simulink model "Ford_T3T6_ArchCnctnDigrm"  (R2016b)
settings: Solver=FixedStepDiscrete  StartTime=0.0  StopTime=10.0  RelTol=1e-3  EnableMultiTasking=on
libraries: canmsglib x15
(part 8 of 15)

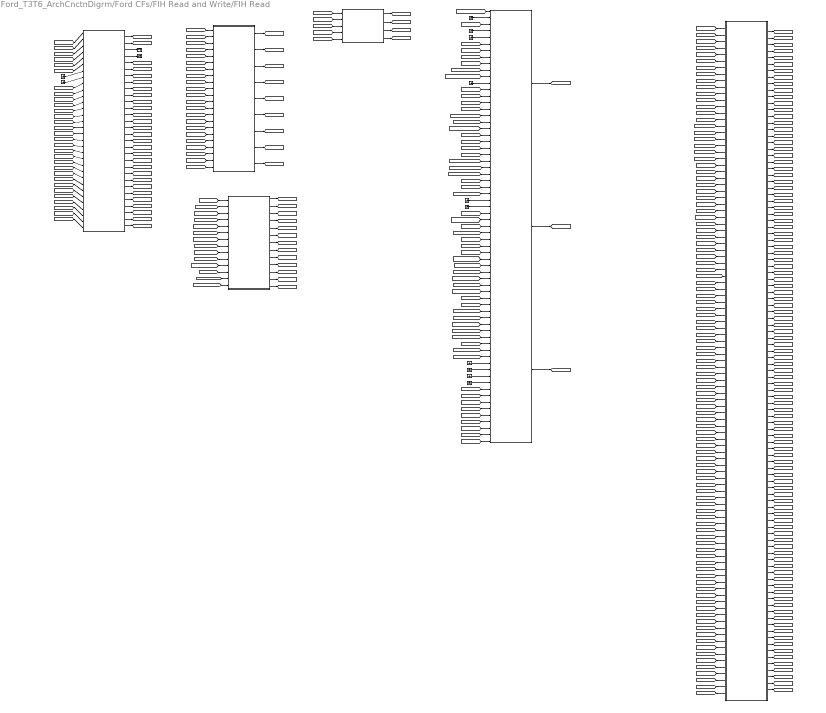
== system Ford_T3T6_ArchCnctnDigrm/Ford CFs/FIH Read and Write/FIH Read ==
  note: ASIL B FIH
  note: ASIL B FIH
  note: ASIL B FIH
  note: ASIL B FIH
  note: ASIL B FIH
  note: ASIL B FIH
  note: FIH_Read_Signal_Status
  note: Enable Disable Feature via DID
  note: Missing in component Req
  note: Bit 2
  note: Status 2 Bit 0
  note: Bit 3
  note: Bit 1
  note: Bit 0
  note: Bit31
  note: Bit24
  note: MM092
  note: Status 2
      | Bit 0 AccelPedalPosValid
      | Bit 1 EngineRPMValid
      | Bit 2 GearLeverPosValid
      | Bit 3 IgnitionStatusValid
      | Bit 4 LSMCBrakeSupportValid
      | Bit 5 PAMStatusValid
      | Bit 6 TBAAvailableValid
      | Bit 7 TBACancelRequestValid
      | Bit 8 TBAEnableValid
      | Bit 9 TBAHitchAngleValid
      | Bit 10 TBAHitchRateValid
      | Bit 11 TBAKnobPositionValid
      | Bit 12 TBAKnobValid
      | Bit 13 TBAMeasurementValid
      | Bit 14 TBATargetValid
      | Bit 15 TBATrackStateValid
      | Bit 16 TBAYawRateValid
      | Bit 17 TBAReverseValid
      | Bit 18 TBAModeRequestValid
      | Bit 19 BrakePedalValid
      | Bit 20-31 NOT USED
  note: Status 1
      | Bit 0 VehicleSpeedValid
      | Bit 1 BrakeTorqueValid
      | Bit 2 VertAccelValid
      | Bit 3 FLWheelCountDirValid
      | Bit 4 FLWheelSpeedValid
      | Bit 5 FRWheelCountDirValid
      | Bit 6 FRWheelSpeedValid
      | Bit 7 LA_IPMAValid
      | Bit 8 LatAccelValid
      | Bit 9 LATCTL_IPMAValid
      | Bit 10 SDMChassisValid
      | Bit 11 PropTorqueValid
      | Bit 12 ReverseGearValid
      | Bit 13 RLWheelCountDirValid
      | Bit 14 RLWheelSpeedValid
      | Bit 15 RRWheelCountDirValid
      | Bit 16 RRWheelSpeedValid
      | Bit 17 SPAOffsetValid
      | Bit 18 TurnSignalValid
      | Bit 19 FilteredVehicleSpeedValid
      | Bit 20 YawRateValid
      | Bit 21 YawRateRawValid
      | Bit 22 YawStabilityValid
      | Bit 23 LongAccelValid
      | Bit 24 ABS_ESC_StatusValid
      | Bit 25 ESA_IPCValid
      | Bit 26 ESA_IPMAValid
      | Bit 27 VehicleSpeedOverGroundValid
      | Bit 28 SPAVelocityValid
      | Bit 29 RelativeSPAValid
      | Bit 30 InputTorqueRawValid
      | Bit 31 AppliedFinalMotorTorqueValid
  note: Add FIH_Read_TBA_EAC_Status()
  note: Add FIH_Read_TBA_EAC_Status() EAC_Status
      | (ExtAgCtrlStsInt)
  note: FIH_Read_APA_Torque_Filtered() APA_Torque_Filtered
      | FIH_Read_EngineSize() EngineTorqueClass
      | FIH_Read_SAPPAngleControlStat1() SAPPAngleControlStat1
      | FIH_Read_SAPPAngleControlStat2() SAPPAngleControlStat2
      | FIH_Read_SAPPAngleControlStat3() SAPPAngleControlStat3
      | FIH_Read_SAPPAngleControlStat4() SAPPAngleControlStat4
      | FIH_Read_SAPPAngleControlStat5() SAPPAngleControlStat5
      | FIH_Read_TBA_EAC_Status() EAC_Status
  note: FIH_Read_EPS_System_Time() SystemTime
      | FIH_Read_WheelBase() VehicleWheelBase
      | FIH_Read_RackPinionRatio() RacktoPinionRatio
      | FIH_Read_VehicleSteeringRatio() VehicleSteeringRatio
      | FIH_Read_EPS_InputTorqueRaw() InputTorqueRaw
      | FIH_Read_EPS_InputTorqueFilt() BCInputTorque
      | FIH_Read_EPS_Assist_Torque() BCAssistTorque
      | FIH_Read_EPS_SteeringAngle() CompensatedSPA
      | FIH_Read_EPS_CompSPA_QF() CompensatedSPAQualityFactor
      | FIH_Read_EPS_ColumnVelocity() SPAVelocity
      | FIH_Read_EPS_VehicleSpeed() FilteredVehicleSpeed
      | FIH_Read_EPS_VehicleSpeed_Raw() VehicleSpeed
      | FIH_Read_TireCircumference() TireCircumference
      | FIH_Read_EPS_Final_Motor_Tq_Rq() RequestedFinalMotorTorque
      | FIH_Read_EPS_Final_Motor_Tq_App() AppliedFinalMotorTorque
      | FIH_Read_EPS_Rel_SteeringAngle() RelativeSPA
      | FIH_Read_EPS_Personalization() SDM_SteeringMode
      | FIH_Read_AngleControlState() INTAngleControlStat1
      | FIH_Read_EPSSystemState() EPSSystemState
      | FIH_Read_MaxAssistanceTorque() MaxAssistanceTorque
  note: To be deleted
  note: To be deleted
  note: CF100
  note: CF100
  note: MMs Does not exist yet
  note: Use FordVehYawRateSnsrIdyHi and FordVehYawRateSnsrIdyLo from MM082
      | and combine them
  note: Should it be FordVehSpdBrkModlVld ??
  note: SDM_SteeringMode
  note: s8p7
  note: U-8
  note: U-32
  note: U-32
  note: U-32
  note: U-32
  note: U-32
  note: U-32
  note: U-32
  note: U-32
  note: U-32
  note: U-16
  note: VehVertComp_A_Actl
  note: GearRvrse_D_Actl
  note: Msg 60A,B,C,D
      | Not available
  note: HSCAN_In4_High
  note: HSCAN_In4_Low
  note: HSCAN_In3_High
  note: HSCAN_In3_Low
  note: HSCAN_In2_High
  note: HSCAN_In2_Low
  note: HSCAN_In1_High
  note: HSCAN_In1_Low
  note: TrlrYaw_W_Actl_D_Qf
  note: TrlrYaw_W_Actl
  note: TrlrIdType_D_Stat
  note: TrlrRvrse_D_Stat
  note: TrlrRvrseMsgTxt_D2_Rq
  note: TrlrHitchYaw_D_Stat
  note: TrlrRvrseEnbl_D2_Stat
  note: TrlrRvrseCancl_B_Rq
  note: TrlrLampCnnct_B_Actl
  note: TrlrAidTrgtId_No_Actl
  note: TrlrHitYaw_AnRate_Actl
  note: TrlrHitchYaw_An_Actl
  note: TrlrBrkActCnnct_B_Actl
  note: HitchToVehAxle_L_Calc
  note: TrlrAxleToBmpr_L_Actl
  note: TrlrAid_D2_Stat
  note: TrlrAidSetup_D2_Rq
  note: TrlrAidEnbl_D2_Rq
  note: TrlrAidMde_D_Rq
  note: TrlrAidCtl_U_RqDrv
  note: TrlrAidSwtch_D_RqDrv
  note: TrlrId_No_Actl
  note: TrlrHitYaw_AnRate_Actl
  note: msg45A
  note: TrlrAnOffstDir_D_Mem
  note: TrlrAid_An3_Actl
  note: TrlrAidCancl_B_Rq
  note: VehVTrlrAid_B_Avail
  note: Msg 459
  note: TrlrTrgtAcquire_D_Stat
  note: Veh_V_ActlBrk
  note: YawStabilityIndex
  note: u-48
  note: Ford_TrlrSnsId_No_Act
  note: VehYaw_W_Actl
  note: VehYawComp_W_Actl
  note: Ford_VehOverGnd_V_Est
  note: Ford_VehLongComp_A_Actl
  note: Ford_VehLatComp_A_Actl
  note: TurnLghtSwtch_D_Stat
  note: Ford_GearPos_D_Actl
  note: TrnRng_D_Rq
  note: CmbbObjColl_T_Actl
  note: EsaOn_B_Rq
  note: CmbbObjRelLong_V_Actl
  note: CmbbObjRelLat_V_Actl
  note: WhlRl_W_Meas
  note: WhlRotatRl_No_Cnt
  note: WhlDirRl_D_Actl
  note: PrplWhlTot2_Tq_Actl
  note: ApaSys_D_Stat
  note: CmbbObjClass_D_Stat
  note: CmbbObjConfdnc_D_Stat
  note: Ford_LsmcBrkDecel_D_Stat1
  note: LaRefAng_No_Req
  note: LaCurvature_No_Calc
  note: CmbbObjDistLong_L_Actl
  note: CmbbObjDistLat_L_Actl
  note: Change source name
  note: LatCtl_D_Rq
  note: LatCtlPrecision_D_Rq
  note: LatCtlPathOffst_L_Actl
  note: LatCtlPath_An_Actl
  note: LatCtlCurv_NoRate_Actl
  note: LatCtlCurv_No_Actl
  note: GearLvrPos_D_Actl
  note: WhlFr_W_Meas
  note: WhlRotatFr_No_Cnt
  note: WhlDirFr_D_Actl
  note: WhlFl_W_Meas
  note: WhlDirFl_D_Actl
  note: EngAout_N_Actl
  note: StabCtlBrkActv_B_Actl
  note: CmbbBrkDis_B_Actl
  note: CmbbDeny_B_ActlBrk
  note: Ignition_Status1
  note: BpedDrvAppl_D_Qf
  note: BpedDrvAppl_D_Actl
  note: StePinOffst_D_Stat1
  note: StePinOffst_An_Est
  note: AbsActv_B_Actl
  note: BrkTot_Tq_Actl
  note: ApedPosPcActl_D_Qf
  note: ApedPos_Pc_ActlArb
  note: LaRampType_B_Req
  note: LatCtlRng_L_Max
  note: LatCtlRampType_D_Rq
  note: HandsOffCnfm_B_Rq
  note: Called by FIH
  note: Called by FIH
  note: Called by FIH
  note: Called by FIH
  note: LkaActvStats_D2_Req
  note: LdwActvStats_D_Req
  note: LdwActvIntns_D_Req
  note: WhlRotatFl_No_Cnt
  note: EsaEnbl_D2_Rq
  note: TireCircumference
      | mm
      | U-16
      | 1
  note: PDC_InternalStatus
      | Table
      | U-32
      |
      | LDW_InternalStatus
      | Table
      | U-32
      |
      | LKA_InternalStatus
      | Table
      | U-32
      |
      | ANC_InternalStatus
      | Table
      | U-32
      |
      | STDR_InternalStatus
      | Table
      | U-32
      |
      | ESA_InternalStatus
      | Table
      | U-32
      |
      | LATCTL_InternalStatus
      | Table
      | U-32
      |
      | TBA_InternalStatus
      | Table
      | U-32
  note: INTAngleControlStat1
      | Table
      | U-8
      |
      | SAPPAngleControlStat1
      | Table
      | U-8
      |
      | SAPPAngleControlStat2
      | No Units
      | Bool
      |
      | SAPPAngleControlStat3
      | No Units
      | Bool
      |
      | SAPPAngleControlStat4
      | No Units
      | Bool
      |
      | SAPPAngleControlStat5
      | No Units
      | Bool
      |
      | SAPPAngleControlStat6
      | No Units
      | Bool
  note: ANC_Diagnostic_Status
      | Table
      | U-8
      |
      | LDW_Diagnostic_Status
      | Table
      | U-8
  note: From DID
  note: // Read --> The Vehicle Physical Parameters (e.g. Wheelbase, Rack-to-Pinion Ratio, etc.) must be provided by Base EPS to In-House Features via Software
      | Read Functions. In-House Features that require these parameters will request it once during Initialization.
  note: WhlRr_W_Meas
  note: WhlRotatRr_No_Cnt
  note: WhlDirRr_D_Actl
  note: To be deleted
  note: To be deleted
  note: To be deleted
  note: To be deleted
  note: To be deleted
  note: To be deleted
  note: To be deleted
  note: To be deleted
  note: CF100
  note: To be deleted
  note: To be deleted
  note: To be deleted
  note: To be deleted
  note: CF100
  note: MM092
  note: Bit 4
  note: Bit 5
  note: Bit 6
  note: Bit 7
  note: Bit 8
  note: Bit 9
  note: Bit 10
  note: Bit 11
  note: Bit 12
  note: Bit 13
  note: Bit 14
  note: Bit 15
  note: Bit 16
  note: Bit 17
  note: Bit 18
  note: Bit 20
  note: Bit 21
  note: Bit 22
  note: Bit 23
  note: Bit 25
  note: Bit 26
  note: Bit 27
  note: Bit 28
  note: Bit 29
  note: Bit 30
  note: Status 2 Bit 1
  note: Status 2 Bit 2
  note: Status 2 Bit 3
  note: Status 2 Bit 4
  note: Status 2 Bit 5
  note: Status 2 Bit 6
  note: Status 2 Bit 7
  note: Status 2 Bit 8
  note: Status 2 Bit 9
  note: Status 2 Bit 10
  note: Status 2 Bit 11
  note: Status 2 Bit 12
  note: Status 2 Bit 13
  note: Status 2 Bit 14
  note: Status 2 Bit 15
  note: Status 2 Bit 16
  note: Status 2 Bit 17
  note: Status 2 Bit 18
  note: Status 2 Bit 19
  note: Bit 19
  note: Missing in component Req
  note: Missing in component Req
  note: FIH_Read_Signal_Status
  note: FIH_Read_Signal_Status
  note: FIH_Read_Signal_Status
  note: FIH_Read_Signal_Status
  note: FIH_Read_Signal_Status
  note: FIH_Read_Signal_Status
  note: FIH_Read_Signal_Status
  note: FIH_Read_Signal_Status
  note: FIH_Read_Signal_Status
  note: FIH_Read_Signal_Status
  note: FIH_Read_Signal_Status
  note: FIH_Read_Signal_Status
  note: FIH_Read_Signal_Status
  note: FIH_Read_Signal_Status
  note: FIH_Read_Signal_Status
  note: FIH_Read_Signal_Status
  note: FIH_Read_Signal_Status
  note: FIH_Read_Signal_Status
  note: FIH_Read_Signal_Status
  note: FIH_Read_Signal_Status
  note: FIH_Read_Signal_Status
  note: FIH_Read_Signal_Status
  note: FIH_Read_Signal_Status
  note: FIH_Read_Signal_Status
  note: FIH_Read_Signal_Status
  note: FIH_Read_Signal_Status
  note: FIH_Read_Signal_Status
  note: FIH_Read_Signal_Status
  note: FIH_Read_Signal_Status
  note: FIH_Read_Signal_Status
  note: FIH_Read_Signal_Status
  note: Called by FIH
  note: Called by FIH
  CF053A_FordBlaBoxEpsRead : Subsystem  Tag=1.0.X  Description=This function is designed to return information from Nexteer software to the Ford In-House (FIH) software, vie a specified function call.
      settings: AttributesFormatString=Version: %<Tag>
  CF054A_FordBlaBoxCanHiSpdRead : Subsystem  Tag=1.0.X  Description=This function is used by Ford In House (FIH) to read HSCAN values. This function has no outputs, as it is only passing inofrmation to FIH function.
      settings: AttributesFormatString=Version: %<Tag>
  CF056A_FordBlaBoxVldRead : Subsystem  Tag=1.0.X  Description=This function reads diagnostic values into Ford In House (FIH). This function has no outputs, as it is only passing information to FIH features from the EPS.
      settings: AttributesFormatString=Version: %<Tag>
  CF057A_FordBlaBoxDiagcRead : Subsystem  Tag=1.0.X  Description=This function reads diagnostic values into Ford InHouse (FIH) functions. This function has no outputs,as it is only passing information to FIH functions.
      settings: AttributesFormatString=Version: %<Tag>
  CF059A_FordBlaBoxFeatStRead : Subsystem  Tag=1.0.X  Description=The Ford Black Box Feature State Read functional returns information fromNexteer software to the Ford In-House (FIH) software, via a specified function call.
      settings: AttributesFormatString=Version: %<Tag>
  CF062A_FordBlaBoxNvmRead : Subsystem  Tag=1.0.X  Description=This function allows Ford In House features to read from their specific NVM loactions.
      settings: AttributesFormatString=Version: %<Tag>
  Ground{,1..11} (12 alike) : Ground
  Terminator : Terminator
  Terminator1 : Terminator
  tag scope: FIH_ANC_Read_NV_Byte=global, FIH_LA_Read_NV_Byte=global, FIH_PDC_Read_NV_Byte=global, FIH_Read_ANC_Arbiter=global, FIH_Read_ANC_Ext_Diag_Status=global, FIH_Read_ANC_Int_Status_DID=global, FIH_Read_APA_Torque_Filtered=global, FIH_Read_AbsActv_B_Actl=global, FIH_Read_AngleControlState=global, FIH_Read_ApedPosPcActl_D_Qf=global, FIH_Read_ApedPos_Pc_ActlArb=global, FIH_Read_BPR_Activation_Cnt=global, FIH_Read_BpedDrvAppl_Actl=global, FIH_Read_BpedDrvAppl_QF=global, FIH_Read_BrkTot_Tq_Actl=global, FIH_Read_CmbbBrkDis_B_Actl=global, FIH_Read_CmbbDeny_B_ActlBrk=global, FIH_Read_CmbbObjClass_D_Stat=global, FIH_Read_CmbbObjColl_T_Actl=global, FIH_Read_CmbbObjConfdnc_D_Stat=global, FIH_Read_CmbbObjDistLat_L_Actl=global, FIH_Read_CmbbObjDistLong_L_Actl=global, FIH_Read_CmbbObjRelLat_V_Actl=global, FIH_Read_CmbbObjRelLong_V_Actl=global, FIH_Read_EPS_Assist_Torque=global, FIH_Read_EPS_ColumnVelocity=global, FIH_Read_EPS_CompSPA_QF=global, FIH_Read_EPS_Final_Motor_Tq_App=global, FIH_Read_EPS_Final_Motor_Tq_Rq=global, FIH_Read_EPS_InputTorqueFilt=global, FIH_Read_EPS_InputTorqueRaw=global, FIH_Read_EPS_Personalization=global, FIH_Read_EPS_Rel_SteeringAngle=global, FIH_Read_EPS_SteeringAngle=global, FIH_Read_EPS_System_Time=global, FIH_Read_EPS_TireCircumference=global, FIH_Read_EPS_VehicleSpeed=global, FIH_Read_EPS_VehicleSpeed_Raw=global, FIH_Read_ESA_Arbiter=global, FIH_Read_ESA_Int_Status_DID=global, FIH_Read_EngAout_N_Actl=global, FIH_Read_EngineSize=global, FIH_Read_EsaEnbl_D_Rq=global, FIH_Read_EsaOn_B_Rq=global, FIH_Read_FIH_EoL_Config=global, FIH_Read_FIH_Msg_In_1_High=global, FIH_Read_FIH_Msg_In_1_Low=global, FIH_Read_FIH_Msg_In_2_High=global, FIH_Read_FIH_Msg_In_2_Low=global, FIH_Read_FIH_Msg_In_3_High=global, FIH_Read_FIH_Msg_In_3_Low=global, FIH_Read_FIH_Msg_In_4_High=global, FIH_Read_FIH_Msg_In_4_Low=global, FIH_Read_GearLvrPos_D_Actl=global, FIH_Read_GearPosition=global, FIH_Read_GearRvrse_D_Actl=global, FIH_Read_HandsOffCnfm_B_Rq=global, FIH_Read_HitchToVehAxle=global, FIH_Read_Ignition_Status=global, FIH_Read_LATCTL_Arbiter=global, FIH_Read_LATCTL_Int_Status_DID=global, FIH_Read_LDW_Arbiter=global, FIH_Read_LDW_Ext_Diag_Status=global, FIH_Read_LDW_Int_Status_DID=global, FIH_Read_LKA_Arbiter=global, FIH_Read_LKA_Int_Status_DID=global, FIH_Read_LaCurvature_No_Calc=global, FIH_Read_LaRampType_B_Req=global, FIH_Read_LaRefAng_No_Req=global, FIH_Read_LatCtlCurv_NoRate_Actl=global, FIH_Read_LatCtlCurv_No_Actl=global, FIH_Read_LatCtlPathOffst_L_Actl=global, FIH_Read_LatCtlPath_An_Actl=global, FIH_Read_LatCtlPrecision_D_Rq=global, FIH_Read_LatCtlRampType_D_Rq=global, FIH_Read_LatCtlRangeMax=global, FIH_Read_LatCtl_D_Rq=global, FIH_Read_LdwActvIntns_D_Req=global, FIH_Read_LdwActvStats_D_Req=global, FIH_Read_LkaActvStats_D_Req=global, FIH_Read_LsmcBrkDecel_D_Stat=global, FIH_Read_MaxAssistanceTorque=global, FIH_Read_PDCLearning_Arbiter=global, FIH_Read_PDC_Arbiter=global, FIH_Read_PDC_Int_Status_DID=global, FIH_Read_PDC_Service_DID=global, FIH_Read_PrplWhlTot2_Tq_Actl=global, FIH_Read_RackPinionRatio=global, FIH_Read_SAPPAngleControlStat1=global, FIH_Read_SAPPAngleControlStat2=global, FIH_Read_SAPPAngleControlStat3=global, FIH_Read_SAPPAngleControlStat4=global, FIH_Read_SAPPAngleControlStat5=global, FIH_Read_SAPPStatusCoding=global, FIH_Read_STDR_Arbiter=global, FIH_Read_STDR_Int_Status_DID=global, FIH_Read_Signal_Status2=global, FIH_Read_Signal_Status=global, FIH_Read_Signal_Status_PassThru=global, FIH_Read_StabCtlBrkActv_B_Actl=global, FIH_Read_SteMdule_D_Stat=global, FIH_Read_StePinOffst_An_Est=global, FIH_Read_StePinOffst_D_Stat=global, FIH_Read_TBA_EAC_Status=global, FIH_Read_TBA_Int_Status_DID=global, FIH_Read_TSC_Activation_Cnt=global, FIH_Read_TrlrAidCancl_B_Rq=global, FIH_Read_TrlrAidCtl_U_RqDrv=global, FIH_Read_TrlrAidEnbl_D2_Rq=global, FIH_Read_TrlrAidSetup_Rq=global, FIH_Read_TrlrAidSwtch_D_RqDrv=global, FIH_Read_TrlrAidTrgtId=global, FIH_Read_TrlrAid_Angle=global, FIH_Read_TrlrAid_AngleRate=global, FIH_Read_TrlrAid_D2_Stat=global, FIH_Read_TrlrAid_Mode_Rq=global, FIH_Read_TrlrAnOffstDir_Mem=global, FIH_Read_TrlrAxleToBmpr_L_Actl=global, FIH_Read_TrlrBrkActCnnct_B_Actl=global, FIH_Read_TrlrHitYaw_AnRate=global, FIH_Read_TrlrHitchYaw_An=global, FIH_Read_TrlrHitchYaw_Stat=global, FIH_Read_TrlrIdType_Stat=global, FIH_Read_TrlrId_No_Actl=global, FIH_Read_TrlrLampCnnct_B_Actl=global, FIH_Read_TrlrRvrseCancl_Rq=global, FIH_Read_TrlrRvrseEnbl=global, FIH_Read_TrlrRvrseMsgTxt=global, FIH_Read_TrlrRvrseOn_Stat=global, FIH_Read_TrlrSnsId=global, FIH_Read_TrlrTrgtAcquire=global, FIH_Read_TrlrYaw_W=global, FIH_Read_TrlrYaw_W_Qf=global, FIH_Read_TrnRng=global, FIH_Read_TurnLghtSwtch_D_Stat=global, FIH_Read_VehLatComp_A_Actl=global, FIH_Read_VehLongComp_A_Actl=global, FIH_Read_VehOverGnd_V_Est=global, FIH_Read_VehVTrlrAid_B_Avail=global, FIH_Read_VehVertComp=global, FIH_Read_VehYawComp_W_Actl=global, FIH_Read_VehYaw_W_Actl=global, FIH_Read_Veh_V_ActlBrk=global, FIH_Read_VehicleSteeringRatio=global, FIH_Read_WheelBase=global, FIH_Read_WhlDirFl_D_Actl=global, FIH_Read_WhlDirFr_D_Actl=global, FIH_Read_WhlDirRl_D_Actl=global, FIH_Read_WhlDirRr_D_Actl=global, FIH_Read_WhlFl_W_Meas=global, FIH_Read_WhlFr_W_Meas=global, FIH_Read_WhlRl_W_Meas=global, FIH_Read_WhlRr_W_Meas=global, FIH_Read_Whl_Fl_Roll_Cnt=global, FIH_Read_Whl_Fr_Roll_Cnt=global, FIH_Read_Whl_Rl_Roll_Cnt=global, FIH_Read_Whl_Rr_Roll_Cnt=global, FIH_Read_YawStabilityIndex=global, FIH_TBA_Read_NV_Byte=global
  wires:
  [ActvParkAssiTqFild] -> CF053A_FordBlaBoxEpsRead/1(ActvParkAssiTqFild)
  [FordAppldFinalMotTq] -> CF053A_FordBlaBoxEpsRead/2(AppldFinalMotTq)
  [FordBoostCrvAssiTq] -> CF053A_FordBlaBoxEpsRead/3(BoostCrvAssiTq)
  [FordBoostCrvInpTq] -> CF053A_FordBlaBoxEpsRead/4(BoostCrvInpTq)
  [EcuId] -> CF053A_FordBlaBoxEpsRead/5(EcuId)
  [EngTqClass] -> CF053A_FordBlaBoxEpsRead/6(EngTqClass)
  Ground/1 -> CF053A_FordBlaBoxEpsRead/7(ExtAgCtrlSpdVld)
  [VehSpd] -> CF053A_FordBlaBoxEpsRead/9(FildVehSpd)
  [FordCmpdHwPosn] -> CF053A_FordBlaBoxEpsRead/10(FordCmpdHwPosn)
  [FordCmpdHwPosnQlyFac] -> CF053A_FordBlaBoxEpsRead/11(FordCmpdHwPosnQlyFac)
  [FordEpsSysSt] -> CF053A_FordBlaBoxEpsRead/12(FordEpsSysSt)
  [FordMaxAsscTq] -> CF053A_FordBlaBoxEpsRead/13(FordMaxAsscTq)
  [FordRelHwPosn] -> CF053A_FordBlaBoxEpsRead/14(FordRelHwPosn)
  [FordVehTireCircum] -> CF053A_FordBlaBoxEpsRead/15(FordVehTireCircum)
  [HwVel] -> CF053A_FordBlaBoxEpsRead/16(HwVel)
  [IntAgCtrlSt] -> CF053A_FordBlaBoxEpsRead/17(INTAgCtrlStat1)
  [FordInpTqRaw] -> CF053A_FordBlaBoxEpsRead/18(InpTqRaw)
  [RackToPinionRat] -> CF053A_FordBlaBoxEpsRead/19(RackToPinionRat)
  [FordReqdFinalMotTq] -> CF053A_FordBlaBoxEpsRead/20(ReqdFinalMotTq)
  [SelctvDrvgModSteerMod] -> CF053A_FordBlaBoxEpsRead/21(SelctvDrvgModSteerMod)
  [SemiAutParlParkAgCtrlSts1] -> CF053A_FordBlaBoxEpsRead/22(SemiAutParlParkAgCtrlSts1)
  [SemiAutParlParkAgCtrlSts2] -> CF053A_FordBlaBoxEpsRead/23(SemiAutParlParkAgCtrlSts2)
  [SemiAutParlParkAgCtrlSts3] -> CF053A_FordBlaBoxEpsRead/24(SemiAutParlParkAgCtrlSts3)
  [SemiAutParlParkAgCtrlSts4] -> CF053A_FordBlaBoxEpsRead/25(SemiAutParlParkAgCtrlSts4)
  [SemiAutParlParkAgCtrlSts5] -> CF053A_FordBlaBoxEpsRead/26(SemiAutParlParkAgCtrlSts5)
  [FordVehSpd] -> CF053A_FordBlaBoxEpsRead/28(VehSpd)
  [VehSteerRat] -> CF053A_FordBlaBoxEpsRead/29(VehSteerRat)
  [VehWhlBas] -> CF053A_FordBlaBoxEpsRead/30(VehWhlBas)
  [GetRefTmr100MicroSec32bit] -> CF053A_FordBlaBoxEpsRead/32(GetRefTmr100MicroSec32bit)
  CF053A_FordBlaBoxEpsRead/1(FIH_Read_APA_Torque_Filtered) -> [FIH_Read_APA_Torque_Filtered]
  CF053A_FordBlaBoxEpsRead/2(FIH_Read_AngleControlState) -> [FIH_Read_AngleControlState]
  CF053A_FordBlaBoxEpsRead/3(FIH_Read_EACSpeedValid) -> Terminator/1
  CF053A_FordBlaBoxEpsRead/4(FIH_Read_EAC_SPAVelocityValid) -> Terminator1/1
  CF053A_FordBlaBoxEpsRead/5(FIH_Read_EPS_Assist_Torque) -> [FIH_Read_EPS_Assist_Torque]
  CF053A_FordBlaBoxEpsRead/6(FIH_Read_EPS_ColumnVelocity) -> [FIH_Read_EPS_ColumnVelocity]
  CF053A_FordBlaBoxEpsRead/7(FIH_Read_EPS_CompSPA_QF) -> [FIH_Read_EPS_CompSPA_QF]
  CF053A_FordBlaBoxEpsRead/8(FIH_Read_EPS_Final_Motor_Tq_App) -> [FIH_Read_EPS_Final_Motor_Tq_App]
  CF053A_FordBlaBoxEpsRead/9(FIH_Read_EPS_Final_Motor_Tq_Rq) -> [FIH_Read_EPS_Final_Motor_Tq_Rq]
  CF053A_FordBlaBoxEpsRead/10(FIH_Read_EPS_InputTorqueFilt) -> [FIH_Read_EPS_InputTorqueFilt]
  CF053A_FordBlaBoxEpsRead/11(FIH_Read_EPS_InputTorqueRaw) -> [FIH_Read_EPS_InputTorqueRaw]
  CF053A_FordBlaBoxEpsRead/12(FIH_Read_EPS_Personalization) -> [FIH_Read_EPS_Personalization]
  CF053A_FordBlaBoxEpsRead/13(FIH_Read_EPS_Rel_SteeringAngle) -> [FIH_Read_EPS_Rel_SteeringAngle]
  CF053A_FordBlaBoxEpsRead/14(FIH_Read_EPS_SteeringAngle) -> [FIH_Read_EPS_SteeringAngle]
  CF053A_FordBlaBoxEpsRead/15(FIH_Read_EPS_System_Time) -> [FIH_Read_EPS_System_Time]
  CF053A_FordBlaBoxEpsRead/16(FIH_Read_EPS_TireCircumference) -> [FIH_Read_EPS_TireCircumference]
  CF053A_FordBlaBoxEpsRead/17(FIH_Read_EPS_VehicleSpeed) -> [FIH_Read_EPS_VehicleSpeed]
  CF053A_FordBlaBoxEpsRead/18(FIH_Read_EPS_VehicleSpeed_Raw) -> [FIH_Read_EPS_VehicleSpeed_Raw]
  CF053A_FordBlaBoxEpsRead/19(FIH_Read_EngineSize) -> [FIH_Read_EngineSize]
  CF053A_FordBlaBoxEpsRead/20(FIH_Read_MaxAssistanceTorque) -> [FIH_Read_MaxAssistanceTorque]
  CF053A_FordBlaBoxEpsRead/21(FIH_Read_RackPinionRatio) -> [FIH_Read_RackPinionRatio]
  CF053A_FordBlaBoxEpsRead/22(FIH_Read_SAPPAngleControlStat1) -> [FIH_Read_SAPPAngleControlStat1]
  CF053A_FordBlaBoxEpsRead/23(FIH_Read_SAPPAngleControlStat2) -> [FIH_Read_SAPPAngleControlStat2]
  CF053A_FordBlaBoxEpsRead/24(FIH_Read_SAPPAngleControlStat3) -> [FIH_Read_SAPPAngleControlStat3]
  CF053A_FordBlaBoxEpsRead/25(FIH_Read_SAPPAngleControlStat4) -> [FIH_Read_SAPPAngleControlStat4]
  CF053A_FordBlaBoxEpsRead/26(FIH_Read_SAPPAngleControlStat5) -> [FIH_Read_SAPPAngleControlStat5]
  CF053A_FordBlaBoxEpsRead/27(FIH_Read_SteMdule_D_Stat) -> [FIH_Read_SteMdule_D_Stat]
  CF053A_FordBlaBoxEpsRead/28(FIH_Read_VehicleSteeringRatio) -> [FIH_Read_VehicleSteeringRatio]
  CF053A_FordBlaBoxEpsRead/29(FIH_Read_WheelBase) -> [FIH_Read_WheelBase]
  [EcuId] -> CF059A_FordBlaBoxFeatStRead/1(EcuId)
  [FordActvNiblCtrlArbnCmd] -> CF059A_FordBlaBoxFeatStRead/2(FordActvNiblCtrlArbiterCmd)
  [FordActvNiblCtrlEnad] -> CF059A_FordBlaBoxFeatStRead/3(FordActvNiblCtrlEnad)
  [FordBrkPlsRejctnEnad] -> CF059A_FordBlaBoxFeatStRead/4(FordBrkPlsRejctnEnad)
  [FordEvasSteerAssiArbnCmd] -> CF059A_FordBlaBoxFeatStRead/5(FordEvasSteerAssiArbiterCmd)
  [FordEvasSteerAssiEnad] -> CF059A_FordBlaBoxFeatStRead/6(FordEvasSteerAssiEnad)
  [FordLaneCentrAssiEnad] -> CF059A_FordBlaBoxFeatStRead/7(FordLaneCenteringAssiEnad)
  [FordLaneDprtrWarnArbnCmd] -> CF059A_FordBlaBoxFeatStRead/8(FordLaneDprtrWarnArbiterCmd)
  [FordLaneDprtrWarnEnad] -> CF059A_FordBlaBoxFeatStRead/9(FordLaneDprtrWarnEnad)
  [FordLaneKeepAssiArbnCmd] -> CF059A_FordBlaBoxFeatStRead/10(FordLaneKeepingAssiArbiterCmd)
  [FordLaneKeepAssiEnad] -> CF059A_FordBlaBoxFeatStRead/11(FordLaneKeepingAssiEnad)
  [FordLatCtrlArbnCmd] -> CF059A_FordBlaBoxFeatStRead/12(FordLatCtrlArbiterCmd)
  [FordPullDriftCmpArbnCmd] -> CF059A_FordBlaBoxFeatStRead/13(FordPullDriftCmpArbiterCmd)
  [FordPullDriftCmpEnad] -> CF059A_FordBlaBoxFeatStRead/14(FordPullDriftCmpEnad)
  [FordPullDriftCmpLrngArbnCmd] -> CF059A_FordBlaBoxFeatStRead/15(FordPullDriftCmpLrngArbiterCmd)
  [FordResrchFctEnad] -> CF059A_FordBlaBoxFeatStRead/16(FordResrchFctEnad)
  [FordSteerDstbcRejctnArbnCmd] -> CF059A_FordBlaBoxFeatStRead/17(FordSteerTqDstbcRejctnArbiterCmd)
  [FordTqSteerCmpEnad] -> CF059A_FordBlaBoxFeatStRead/18(FordTqSteerCmpEnad)
  [FordTrfcJamAssiEnad] -> CF059A_FordBlaBoxFeatStRead/19(FordTrfcJamAssiEnad)
  [FordTrlrBackupAssi5WhlEnad] -> CF059A_FordBlaBoxFeatStRead/20(FordTrlrBackupAssi5WhlEnad)
  [FordTrlrBackupAssiEnad] -> CF059A_FordBlaBoxFeatStRead/21(FordTrlrBackupAssiEnad)
  [FordTrlrBackupAssiTRGEnad] -> CF059A_FordBlaBoxFeatStRead/22(FordTrlrBackupAssiTRGEnad)
  CF059A_FordBlaBoxFeatStRead/1(FIH_Read_ANC_Arbiter) -> [FIH_Read_ANC_Arbiter]
  CF059A_FordBlaBoxFeatStRead/2(FIH_Read_ESA_Arbiter) -> [FIH_Read_ESA_Arbiter]
  CF059A_FordBlaBoxFeatStRead/3(FIH_Read_FIH_EoL_Config) -> [FIH_Read_FIH_EoL_Config]
  CF059A_FordBlaBoxFeatStRead/4(FIH_Read_LATCTL_Arbiter) -> [FIH_Read_LATCTL_Arbiter]
  CF059A_FordBlaBoxFeatStRead/5(FIH_Read_LDW_Arbiter) -> [FIH_Read_LDW_Arbiter]
  CF059A_FordBlaBoxFeatStRead/6(FIH_Read_LKA_Arbiter) -> [FIH_Read_LKA_Arbiter]
  CF059A_FordBlaBoxFeatStRead/7(FIH_Read_PDCLearning_Arbiter) -> [FIH_Read_PDCLearning_Arbiter]
  CF059A_FordBlaBoxFeatStRead/8(FIH_Read_PDC_Arbiter) -> [FIH_Read_PDC_Arbiter]
  CF059A_FordBlaBoxFeatStRead/9(FIH_Read_STDR_Arbiter) -> [FIH_Read_STDR_Arbiter]
  [FordActvNiblCtrlDiagcSts] -> CF057A_FordBlaBoxDiagcRead/1(ANCDiagcStsInt)
  [FordWrSrvActvNiblCmpIntSts] -> CF057A_FordBlaBoxDiagcRead/2(ANCIntSts)
  [FordWrSrvBrkPlsRednActvnCntr] -> CF057A_FordBlaBoxDiagcRead/3(BPRActvnCntInt)
  [FordWrSrvEvasSteerAssiIntSts] -> CF057A_FordBlaBoxDiagcRead/4(ESAIntSts)
  [EcuId] -> CF057A_FordBlaBoxDiagcRead/5(EcuId)
  [FordWrSrvLatCtrlIntSts] -> CF057A_FordBlaBoxDiagcRead/6(LATCTLIntSts)
  [FordSrvLaneDprtrWarnDiagcSts] -> CF057A_FordBlaBoxDiagcRead/7(LDWDiagcStsInt)
  [FordWrSrvLaneDprtrWarnIntSts] -> CF057A_FordBlaBoxDiagcRead/8(LDWIntSts)
  [FordWrSrvLaneKeepAssiIntSts] -> CF057A_FordBlaBoxDiagcRead/9(LKAIntSts)
  [FordWrSrvPullDriftCmpIntSts] -> CF057A_FordBlaBoxDiagcRead/10(PDCIntSts)
  [FordWrSrvSteerTqDstbcRejctnIntSts] -> CF057A_FordBlaBoxDiagcRead/11(STDRIntSts)
  [SrvPullDriftCmpRstVal] -> CF057A_FordBlaBoxDiagcRead/12(SrvPDCRstValInt)
  [FordWrSrvTrlrBackupAssiIntSts] -> CF057A_FordBlaBoxDiagcRead/13(TBAIntSts)
  [FordWrSrvTqSteerCmpActvnCntr] -> CF057A_FordBlaBoxDiagcRead/14(TSCActvnCntInt)
  CF057A_FordBlaBoxDiagcRead/1(FIH_Read_ANC_Ext_Diag_Status) -> [FIH_Read_ANC_Ext_Diag_Status]
  CF057A_FordBlaBoxDiagcRead/2(FIH_Read_ANC_Int_Status_DID) -> [FIH_Read_ANC_Int_Status_DID]
  CF057A_FordBlaBoxDiagcRead/3(FIH_Read_BPR_Activation_Cnt) -> [FIH_Read_BPR_Activation_Cnt]
  CF057A_FordBlaBoxDiagcRead/4(FIH_Read_ESA_Int_Status_DID) -> [FIH_Read_ESA_Int_Status_DID]
  CF057A_FordBlaBoxDiagcRead/5(FIH_Read_LATCTL_Int_Status_DID) -> [FIH_Read_LATCTL_Int_Status_DID]
  CF057A_FordBlaBoxDiagcRead/6(FIH_Read_LDW_Ext_Diag_Status) -> [FIH_Read_LDW_Ext_Diag_Status]
  CF057A_FordBlaBoxDiagcRead/7(FIH_Read_LDW_Int_Status_DID) -> [FIH_Read_LDW_Int_Status_DID]
  CF057A_FordBlaBoxDiagcRead/8(FIH_Read_LKA_Int_Status_DID) -> [FIH_Read_LKA_Int_Status_DID]
  CF057A_FordBlaBoxDiagcRead/9(FIH_Read_PDC_Int_Status_DID) -> [FIH_Read_PDC_Int_Status_DID]
  CF057A_FordBlaBoxDiagcRead/10(FIH_Read_PDC_Service_DID) -> [FIH_Read_PDC_Service_DID]
  CF057A_FordBlaBoxDiagcRead/11(FIH_Read_STDR_Int_Status_DID) -> [FIH_Read_STDR_Int_Status_DID]
  CF057A_FordBlaBoxDiagcRead/12(FIH_Read_TBA_Int_Status_DID) -> [FIH_Read_TBA_Int_Status_DID]
  CF057A_FordBlaBoxDiagcRead/13(FIH_Read_TSC_Activation_Cnt) -> [FIH_Read_TSC_Activation_Cnt]
  [FordVehAccrPedlPosnStsVld] -> CF056A_FordBlaBoxVldRead/1(APedlPosVld)
  Ground2/1 -> CF056A_FordBlaBoxVldRead/2(AbsActvVld)
  [FordAppldFinalMotTqVld] -> CF056A_FordBlaBoxVldRead/3(AppldFinalMotTqVld)
  Ground3/1 -> CF056A_FordBlaBoxVldRead/4(BrkTqArbnVld)
  Ground4/1 -> CF056A_FordBlaBoxVldRead/5(BrkTqDrvVld)
  [FordVehBrkTqVld] -> CF056A_FordBlaBoxVldRead/6(BrkTqVld)
  [EcuId] -> CF056A_FordBlaBoxVldRead/7(EcuId)
  [FordVehEngSpdVld] -> CF056A_FordBlaBoxVldRead/8(EngRPMVld)
  [FordVehAbsEscStsVld] -> CF056A_FordBlaBoxVldRead/9(EsaAbsVld)
  [FordVehEvasSteerAssiReqVld] -> CF056A_FordBlaBoxVldRead/10(EsaIpcVld)
  [FordVehEvasSteerAssiImgProcrModlAVld] -> CF056A_FordBlaBoxVldRead/11(EsaIpmAVld)
  Ground5/1 -> CF056A_FordBlaBoxVldRead/12(EscActvVld)
  [FihMsgInp1Vld] -> CF056A_FordBlaBoxVldRead/13(FihMsgInp1Vld)
  [FihMsgInp2Vld] -> CF056A_FordBlaBoxVldRead/14(FihMsgInp2Vld)
  [FihMsgInp3Vld] -> CF056A_FordBlaBoxVldRead/15(FihMsgInp3Vld)
  [FihMsgInp4Vld] -> CF056A_FordBlaBoxVldRead/16(FihMsgInp4Vld)
  [FordVehFrntLeWhlCntrDirVld] -> CF056A_FordBlaBoxVldRead/17(FrntLeWhlCntDirVld)
  [FordVehFrntLeWhlSpdVld] -> CF056A_FordBlaBoxVldRead/18(FrntLeWhlSpdVld)
  [FordVehFrntRiWhlCntrDirVld] -> CF056A_FordBlaBoxVldRead/19(FrntRiWhlCntDirVld)
  [FordVehFrntRiWhlSpdVld] -> CF056A_FordBlaBoxVldRead/20(FrntRiWhlSpdVld)
  [FordVehGearLvrPosnVld] -> CF056A_FordBlaBoxVldRead/21(GearLvrPosVld)
  [FordVehIgnStsVld] -> CF056A_FordBlaBoxVldRead/22(IgnStsVld)
  [FordInpTqRawVld] -> CF056A_FordBlaBoxVldRead/23(InpTqRawVld)
  [FordVehLatCtrlImgProcrModlAVld] -> CF056A_FordBlaBoxVldRead/24(LATCTLIpmAVld)
  [FordVehLoSpdMtnCtrlBrkSprtVld] -> CF056A_FordBlaBoxVldRead/25(LSMCBrkSprtVld)
  [FordVehLaneAssiImgProcgModlAVld] -> CF056A_FordBlaBoxVldRead/26(LaIpmAVld)
  [FordVehLatACmpdVld] -> CF056A_FordBlaBoxVldRead/27(LatAVld)
  [FordVehLgtACmpdVld] -> CF056A_FordBlaBoxVldRead/28(LongAVld)
  [FordVehParkAidModlStsVld] -> CF056A_FordBlaBoxVldRead/29(PamStsVld)
  Ground6/1 -> CF056A_FordBlaBoxVldRead/30(ParkAidMsgVld)
  Ground7/1 -> CF056A_FordBlaBoxVldRead/31(ParkAidSnsrVld)
  [FordVehPrpnWhlTqVld] -> CF056A_FordBlaBoxVldRead/32(PropTqVld)
  [FordVehReLeWhlCntrDirVld] -> CF056A_FordBlaBoxVldRead/33(ReLeWhlCntDirVld)
  [FordVehReLeWhlSpdVld] -> CF056A_FordBlaBoxVldRead/34(ReLeWhlSpdVld)
  [FordVehReRiWhlCntrDirVld] -> CF056A_FordBlaBoxVldRead/35(ReRiWhlCntDirVld)
  [FordVehReRiWhlSpdVld] -> CF056A_FordBlaBoxVldRead/36(ReRiWhlSpdVld)
  [FordRelHwPosnVld] -> CF056A_FordBlaBoxVldRead/37(RelSpaVld)
  [FordVehGearRvsStsVld] -> CF056A_FordBlaBoxVldRead/38(RvsGearVld)
  [FordVehSelDrvModChassisVld] -> CF056A_FordBlaBoxVldRead/39(SdmChassisVld)
  [FordVehSteerPinionAgOffsVld] -> CF056A_FordBlaBoxVldRead/40(SpaOffsVld)
  [FordHwVelVld] -> CF056A_FordBlaBoxVldRead/41(SpaVelVld)
  [FordVehTrlrBackupAssiAvlVld] -> CF056A_FordBlaBoxVldRead/42(TrlrBackupAssiAvlVld)
  [FordVehTrlrAidCanclReqVld] -> CF056A_FordBlaBoxVldRead/43(TrlrBackupAssiCnclReqVld)
  [FordVehTrlrBackUpAssiEnaVld] -> CF056A_FordBlaBoxVldRead/44(TrlrBackupAssiEnaVld)
  [FordVehTrlrHitchAgVld] -> CF056A_FordBlaBoxVldRead/45(TrlrBackupAssiHitchAgVld)
  [FordVehTrlrHitchRateVld] -> CF056A_FordBlaBoxVldRead/46(TrlrBackupAssiHitchRateVld)
  [FordVehTrlrAidKnobPosnVld] -> CF056A_FordBlaBoxVldRead/47(TrlrBackupAssiKnobPosnVld)
  [FordVehTrlrAidKnobStsVld] -> CF056A_FordBlaBoxVldRead/48(TrlrBackupAssiKnobVld)
  [FordVehTrlrBackupAssiMeasVld] -> CF056A_FordBlaBoxVldRead/49(TrlrBackupAssiMeasurmentVld)
  [FordVehTrlrAidModReqVld] -> CF056A_FordBlaBoxVldRead/50(TrlrBackupAssiModReqVld)
  [FordVehTrlrBackUpAssiRvsVld] -> CF056A_FordBlaBoxVldRead/51(TrlrBackupAssiRvsVld)
  [FordVehTrlrTarVld] -> CF056A_FordBlaBoxVldRead/52(TrlrBackupAssiTarVld)
  [FordVehTrlrAidTrakgStVld] -> CF056A_FordBlaBoxVldRead/53(TrlrBackupAssiTrackStVld)
  [TrlrBackupAssiYawRateVld] -> CF056A_FordBlaBoxVldRead/54(TrlrBackupAssiYawRateVld)
  Ground8/1 -> CF056A_FordBlaBoxVldRead/55(TrlrBrkCnctnVld)
  Ground9/1 -> CF056A_FordBlaBoxVldRead/56(TrlrLampCnctnVld)
  Ground10/1 -> CF056A_FordBlaBoxVldRead/57(TrlrTarOffsVld)
  Ground11/1 -> CF056A_FordBlaBoxVldRead/58(TrlrTarToBmpVld)
  [FordVehTurnSigVld] -> CF056A_FordBlaBoxVldRead/59(TurnSigVld)
  [FordVehSpdOverGndVld] -> CF056A_FordBlaBoxVldRead/60(VehSpdOverGndVld)
  [VehSpdVld] -> CF056A_FordBlaBoxVldRead/61(VehSpdVld)
  [FordVehYawRateRawVld] -> CF056A_FordBlaBoxVldRead/62(YawRateRawVld)
  [FordVehYawRateRawVld] -> CF056A_FordBlaBoxVldRead/63(YawRateVld)
  [FordVehYawStabyVld] -> CF056A_FordBlaBoxVldRead/64(YawStabyVld)
  CF056A_FordBlaBoxVldRead/1(FIH_Read_Signal_Status) -> [FIH_Read_Signal_Status]
  CF056A_FordBlaBoxVldRead/2(FIH_Read_Signal_Status2) -> [FIH_Read_Signal_Status2]
  CF056A_FordBlaBoxVldRead/3(FIH_Read_Signal_Status_PassThru) -> [FIH_Read_Signal_Status_PassThru]
  [EcuId] -> CF054A_FordBlaBoxCanHiSpdRead/1(EcuId)
  [FordVehAccrPedlPosnStsRaw] -> CF054A_FordBlaBoxCanHiSpdRead/2(FordAccrPedlPosnSts)
  [FordVehAccrPedlPosnStsQlyFacRaw] -> CF054A_FordBlaBoxCanHiSpdRead/3(FordAccrPedlPosnStsQlyFac)
  [FordVehActBrkTqRaw] -> CF054A_FordBlaBoxCanHiSpdRead/4(FordActBrkTq)
  [FordVehAbsActv] -> CF054A_FordBlaBoxCanHiSpdRead/5(FordAntilckBrkgSysActv)
  [FordVehSteerPinionAgOffsRaw] -> CF054A_FordBlaBoxCanHiSpdRead/6(FordAntilckBrkgSysElectcStabyCtrlSpaOffs)
  [FordVehSteerPinionOffsStsRaw] -> CF054A_FordBlaBoxCanHiSpdRead/7(FordAntilckBrkgSysElectcStabyCtrlSpaOffsSts)
  [FordVehBrkPedlAppld] -> CF054A_FordBlaBoxCanHiSpdRead/8(FordBrkPedlAppld)
  [FordVehBrkPedlAppldQlyFac] -> CF054A_FordBlaBoxCanHiSpdRead/9(FordBrkPedlAppldQlyFac)
  [FordVehIgnSts] -> CF054A_FordBlaBoxCanHiSpdRead/10(FordCanIgnSts)
  [FordVehCllsnMtgtnByBrkgDenied] -> CF054A_FordBlaBoxCanHiSpdRead/11(FordCllsnMtgtnByBrkgDenied)
  [FordVehCllsnMtgtnByBrkgDisad] -> CF054A_FordBlaBoxCanHiSpdRead/12(FordCllsnMtgtnByBrkgDisad)
  [FordVehEscActv] -> CF054A_FordBlaBoxCanHiSpdRead/13(FordElectcStabyCtrlActv)
  [FordVehEngSpdRaw] -> CF054A_FordBlaBoxCanHiSpdRead/14(FordEngSpd)
  [FordVehEvasSteerAssiEnadReqRaw] -> CF054A_FordBlaBoxCanHiSpdRead/15(FordEvasSteerAssiEnaReq)
  [FordVehFrntLeWhlDirRaw] -> CF054A_FordBlaBoxCanHiSpdRead/16(FordFrntLeWhlDir)
  [FordVehFrntLeWhlRollgCntr] -> CF054A_FordBlaBoxCanHiSpdRead/17(FordFrntLeWhlRollgCnt)
  [FordVehFrntLeWhlSpdRaw] -> CF054A_FordBlaBoxCanHiSpdRead/18(FordFrntLeWhlSpd)
  [FordVehFrntRiWhlDirRaw] -> CF054A_FordBlaBoxCanHiSpdRead/19(FordFrntRiWhlDir)
  [FordVehFrntRiWhlRollgCntr] -> CF054A_FordBlaBoxCanHiSpdRead/20(FordFrntRiWhlRollgCnt)
  [FordVehFrntRiWhlSpdRaw] -> CF054A_FordBlaBoxCanHiSpdRead/21(FordFrntRiWhlSpd)
  [FordVehGearLvrPosnPassd] -> CF054A_FordBlaBoxCanHiSpdRead/22(FordGearLvrPosn)
  [FordVehLaneDetnWarnInten] -> CF054A_FordBlaBoxCanHiSpdRead/23(FordLaneDprtrWarnInten)
  [FordVehLaneDetnWarnSts] -> CF054A_FordBlaBoxCanHiSpdRead/24(FordLaneDprtrWarnSts)
  [FordVehLaneKeepSysSts] -> CF054A_FordBlaBoxCanHiSpdRead/25(FordLaneKeepAssiSts)
  [FordVehLatCtrlCrvtRaw] -> CF054A_FordBlaBoxCanHiSpdRead/26(FordLatCtrlCrvt)
  [FordVehLatCtrlCrvtRateRaw] -> CF054A_FordBlaBoxCanHiSpdRead/27(FordLatCtrlCrvtRate)
  [FordVehLatCtrlHandsOffDetnTqStimlsReq] -> CF054A_FordBlaBoxCanHiSpdRead/28(FordLatCtrlHandsOffDetnTqStimlsReq)
  [FordVehLatCtrlPahRaw] -> CF054A_FordBlaBoxCanHiSpdRead/29(FordLatCtrlPah)
  [FordVehLatCtrlPahOffsRaw] -> CF054A_FordBlaBoxCanHiSpdRead/30(FordLatCtrlPahOffs)
  [FordVehLatCtrlPrcsn] -> CF054A_FordBlaBoxCanHiSpdRead/31(FordLatCtrlPrcsn)
  [FordVehLatCtrlRampTyp] -> CF054A_FordBlaBoxCanHiSpdRead/32(FordLatCtrlRampTyp)
  [FordVehLatCtrlReq] -> CF054A_FordBlaBoxCanHiSpdRead/33(FordLatCtrlReq)
  [FordVehLatCtrlRingMax] -> CF054A_FordBlaBoxCanHiSpdRead/34(FordLatCtrlRngMax)
  [FordVehCllsnMtgtnByBrkgLatDstRaw] -> CF054A_FordBlaBoxCanHiSpdRead/35(FordLatDst)
  [FordVehCllsnMtgtnByBrkgLgtDstRaw] -> CF054A_FordBlaBoxCanHiSpdRead/36(FordLgtDst)
  [FordVehLaneKeepSysCrvtRaw] -> CF054A_FordBlaBoxCanHiSpdRead/37(FordLksCrvt)
  [FordVehLaneKeepSysRampTyp] -> CF054A_FordBlaBoxCanHiSpdRead/38(FordLksRampTyp)
  [FordVehLaneKeepSysReqdAgRaw] -> CF054A_FordBlaBoxCanHiSpdRead/39(FordLksReqdAg)
  [FordVehLoSpdMtnCtrlBrkSprtStsRaw] -> CF054A_FordBlaBoxCanHiSpdRead/40(FordLsmcBrkSprtSts)
  [FordVehCllsnMtgtnByBrkgObjDataConfLvlRaw] -> CF054A_FordBlaBoxCanHiSpdRead/41(FordObjDataConfLvl)
  [FordVehCllsnMtgtnByBrkgObjTypClassnRaw] -> CF054A_FordBlaBoxCanHiSpdRead/42(FordObjTypClassn)
  [FordVehParkAidModlSysSt] -> CF054A_FordBlaBoxCanHiSpdRead/43(FordPamSysSt)
  [FordVehPrpnWhlTqRaw] -> CF054A_FordBlaBoxCanHiSpdRead/44(FordPrpnWhlTq)
  [FordVehTrlrHitchYawSts] -> CF054A_FordBlaBoxCanHiSpdRead/45(FordRcmTrlrAgSts)
  [FordVehReLeWhlDirRaw] -> CF054A_FordBlaBoxCanHiSpdRead/46(FordReLeWhlDir)
  [FordVehReLeWhlRollgCntr] -> CF054A_FordBlaBoxCanHiSpdRead/47(FordReLeWhlRollgCnt)
  [FordVehReLeWhlSpdRaw] -> CF054A_FordBlaBoxCanHiSpdRead/48(FordReLeWhlSpd)
  [FordVehReRiWhlDirRaw] -> CF054A_FordBlaBoxCanHiSpdRead/49(FordReRiWhlDir)
  [FordVehReRiWhlRollgCntr] -> CF054A_FordBlaBoxCanHiSpdRead/50(FordReRiWhlRollgCnt)
  [FordVehReRiWhlSpdRaw] -> CF054A_FordBlaBoxCanHiSpdRead/51(FordReRiWhlSpd)
  [FordVehCllsnMtgtnByBrkgRelLatVelRaw] -> CF054A_FordBlaBoxCanHiSpdRead/52(FordRelLatVel)
  [FordVehCllsnMtgtnByBrkgRelLgtVelRaw] -> CF054A_FordBlaBoxCanHiSpdRead/53(FordRelLgtVel)
  [FordVehEvasSteerAssiReq] -> CF054A_FordBlaBoxCanHiSpdRead/54(FordReqdEvasSteerAssiMod)
  [FordVehCllsnMtgtnByBrkgTiToCllsnRaw] -> CF054A_FordBlaBoxCanHiSpdRead/55(FordTiToCllsn)
  [FordVehTrlrAidAcqSts] -> CF054A_FordBlaBoxCanHiSpdRead/56(FordTrlrAidAcqFihTadIdSts)
  [FordVehTrlrAidAvlRaw] -> CF054A_FordBlaBoxCanHiSpdRead/57(FordTrlrAidAvl)
  [FordVehTrlrAidCnclReq] -> CF054A_FordBlaBoxCanHiSpdRead/58(FordTrlrAidCnclReq)
  [FordVehTrlrAidHitchAg] -> CF054A_FordBlaBoxCanHiSpdRead/59(FordTrlrAidHitchAg)
  [FordVehTrlrAgOffsDirRawPassd] -> CF054A_FordBlaBoxCanHiSpdRead/60(FordTrlrAidHitchAgMemMgnData)
  [FordVehTrlrHitchAgRateRaw] -> CF054A_FordBlaBoxCanHiSpdRead/61(FordTrlrAidHitchAgRate)
  [FordVehTrlrAidIdnNrRawPassd] -> CF054A_FordBlaBoxCanHiSpdRead/62(FordTrlrAidIdNr)
  [FordVehTrlrAidKnobBtn] -> CF054A_FordBlaBoxCanHiSpdRead/63(FordTrlrAidKnobBtn)
  [FordVehTrlrAidKnobPosn] -> CF054A_FordBlaBoxCanHiSpdRead/64(FordTrlrAidKnobPosn)
  [FordVehTrlrAidModReq] -> CF054A_FordBlaBoxCanHiSpdRead/65(FordTrlrAidModReq)
  [FordVehTrlrEnaReqRawPassd] -> CF054A_FordBlaBoxCanHiSpdRead/66(FordTrlrAidOnReq)
  [FordVehTrlrAidSetUpRawPassd] -> CF054A_FordBlaBoxCanHiSpdRead/67(FordTrlrAidSetupReq)
  [FordVehTrlrAidTrakgSt] -> CF054A_FordBlaBoxCanHiSpdRead/68(FordTrlrAidTrakSt)
  [FordVehTrlrAxleToBmpRaw] -> CF054A_FordBlaBoxCanHiSpdRead/69(FordTrlrAxleToBmp)
  [FordVehTrlrBallToAxle] -> CF054A_FordBlaBoxCanHiSpdRead/70(FordTrlrBallToAxle)
  [FordVehTrlrBrkCnctnStsRaw] -> CF054A_FordBlaBoxCanHiSpdRead/71(FordTrlrBrkCnctnSts)
  [FordVehTrlrHitchYawAgRaw] -> CF054A_FordBlaBoxCanHiSpdRead/72(FordTrlrHitchAg)
  [FordVehTrlrHitchAgRateRaw] -> CF054A_FordBlaBoxCanHiSpdRead/73(FordTrlrHitchAgRate)
  [FordVehTrlrAidIdnVal] -> CF054A_FordBlaBoxCanHiSpdRead/74(FordTrlrIdVal)
  [FordVehTrlrLampCnctnStsRaw] -> CF054A_FordBlaBoxCanHiSpdRead/75(FordTrlrLampCnctnSts)
  [FordVehTrlrRvsCnclReqRawPassd] -> CF054A_FordBlaBoxCanHiSpdRead/76(FordTrlrRvsGuidcCnclReq)
  [FordVehTrlrRvsEnaRawPassd] -> CF054A_FordBlaBoxCanHiSpdRead/77(FordTrlrRvsGuidcEna)
  [FordVehTrlrRvsMsgTxtReqRawPassd] -> CF054A_FordBlaBoxCanHiSpdRead/78(FordTrlrRvsGuidcMsgTxtReq)
  [FordVehTrlrAidTrlrRvsGuidcStsPassd] -> CF054A_FordBlaBoxCanHiSpdRead/79(FordTrlrRvsGuidcSts)
  [FordVehTrlrIdnTypRawPassd] -> CF054A_FordBlaBoxCanHiSpdRead/80(FordTrlrTyp)
  [FordVehTrlrYawRateRaw] -> CF054A_FordBlaBoxCanHiSpdRead/81(FordTrlrYawRateAct)
  [FordVehTrlrYawRateQlyFac] -> CF054A_FordBlaBoxCanHiSpdRead/82(FordTrlrYawRateQlyFac)
  [FordVehTrsmDesGearRawPassd] -> CF054A_FordBlaBoxCanHiSpdRead/83(FordTrsmDesGearShift)
  [FordVehGearPosnRawPassd] -> CF054A_FordBlaBoxCanHiSpdRead/84(FordTrsmGearPosn)
  [FordVehTurnSigSwtStsRaw] -> CF054A_FordBlaBoxCanHiSpdRead/85(FordTurnSigSwtSts)
  [FordVehBlaBoxInp1HiPart] -> CF054A_FordBlaBoxCanHiSpdRead/86(FordVehBBMsgInp1HiPart)
  [FordVehBlaBoxInp1LoPart] -> CF054A_FordBlaBoxCanHiSpdRead/87(FordVehBBMsgInp1LoPart)
  [FordVehBlaBoxInp2HiPart] -> CF054A_FordBlaBoxCanHiSpdRead/88(FordVehBBMsgInp2HiPart)
  [FordVehBlaBoxInp2LoPart] -> CF054A_FordBlaBoxCanHiSpdRead/89(FordVehBBMsgInp2LoPart)
  [FordVehBlaBoxInp3HiPart] -> CF054A_FordBlaBoxCanHiSpdRead/90(FordVehBBMsgInp3HiPart)
  [FordVehBlaBoxInp3LoPart] -> CF054A_FordBlaBoxCanHiSpdRead/91(FordVehBBMsgInp3LoPart)
  [FordVehBlaBoxInp4HiPart] -> CF054A_FordBlaBoxCanHiSpdRead/92(FordVehBBMsgInp4HiPart)
  [FordVehBlaBoxInp4LoPart] -> CF054A_FordBlaBoxCanHiSpdRead/93(FordVehBBMsgInp4LoPart)
  [FordVehGearRvsStsRaw] -> CF054A_FordBlaBoxCanHiSpdRead/94(FordVehInRvs)
  [FordVehLgtACmpdRaw] -> CF054A_FordBlaBoxCanHiSpdRead/95(FordVehLatACmpd)
  [FordVehLgtACmpdRaw] -> CF054A_FordBlaBoxCanHiSpdRead/96(FordVehLgtACmpd)
  [FordVehSpdOverGndRaw] -> CF054A_FordBlaBoxCanHiSpdRead/97(FordVehSpdOverGnd)
  [FordVehVertACmpdRaw] -> CF054A_FordBlaBoxCanHiSpdRead/98(FordVehVertARateCmpd)
  [FordVehYawRateRaw] -> CF054A_FordBlaBoxCanHiSpdRead/99(FordVehYawRate)
  [FordVehYawRateCmpdRaw] -> CF054A_FordBlaBoxCanHiSpdRead/100(FordVehYawRateCmpd)
  [Ford_TrlrSnsId_No_Act] -> CF054A_FordBlaBoxCanHiSpdRead/101(FordYawRateSnsrId)
  [FordVehYawStabyRaw] -> CF054A_FordBlaBoxCanHiSpdRead/102(FordYawStaby)
  [FordVehSpdBrkModlRaw] -> CF054A_FordBlaBoxCanHiSpdRead/103(VehSpd)
  CF054A_FordBlaBoxCanHiSpdRead/1(FIH_Read_AbsActv_B_Actl) -> [FIH_Read_AbsActv_B_Actl]
  CF054A_FordBlaBoxCanHiSpdRead/2(FIH_Read_ApedPosPcActl_D_Qf) -> [FIH_Read_ApedPosPcActl_D_Qf]
  CF054A_FordBlaBoxCanHiSpdRead/3(FIH_Read_ApedPos_Pc_ActlArb) -> [FIH_Read_ApedPos_Pc_ActlArb]
  CF054A_FordBlaBoxCanHiSpdRead/4(FIH_Read_BpedDrvAppl_Actl) -> [FIH_Read_BpedDrvAppl_Actl]
  CF054A_FordBlaBoxCanHiSpdRead/5(FIH_Read_BpedDrvAppl_QF) -> [FIH_Read_BpedDrvAppl_QF]
  CF054A_FordBlaBoxCanHiSpdRead/6(FIH_Read_BrkTot_Tq_Actl) -> [FIH_Read_BrkTot_Tq_Actl]
  CF054A_FordBlaBoxCanHiSpdRead/7(FIH_Read_CmbbBrkDis_B_Actl) -> [FIH_Read_CmbbBrkDis_B_Actl]
  CF054A_FordBlaBoxCanHiSpdRead/8(FIH_Read_CmbbDeny_B_ActlBrk) -> [FIH_Read_CmbbDeny_B_ActlBrk]
  CF054A_FordBlaBoxCanHiSpdRead/9(FIH_Read_CmbbObjClass_D_Stat) -> [FIH_Read_CmbbObjClass_D_Stat]
  CF054A_FordBlaBoxCanHiSpdRead/10(FIH_Read_CmbbObjColl_T_Actl) -> [FIH_Read_CmbbObjColl_T_Actl]
  CF054A_FordBlaBoxCanHiSpdRead/11(FIH_Read_CmbbObjConfdnc_D_Stat) -> [FIH_Read_CmbbObjConfdnc_D_Stat]
  CF054A_FordBlaBoxCanHiSpdRead/12(FIH_Read_CmbbObjDistLat_L_Actl) -> [FIH_Read_CmbbObjDistLat_L_Actl]
  CF054A_FordBlaBoxCanHiSpdRead/13(FIH_Read_CmbbObjDistLong_L_Actl) -> [FIH_Read_CmbbObjDistLong_L_Actl]
  CF054A_FordBlaBoxCanHiSpdRead/14(FIH_Read_CmbbObjRelLat_V_Actl) -> [FIH_Read_CmbbObjRelLat_V_Actl]
  CF054A_FordBlaBoxCanHiSpdRead/15(FIH_Read_CmbbObjRelLong_V_Actl) -> [FIH_Read_CmbbObjRelLong_V_Actl]
  CF054A_FordBlaBoxCanHiSpdRead/16(FIH_Read_EngAout_N_Actl) -> [FIH_Read_EngAout_N_Actl]
  CF054A_FordBlaBoxCanHiSpdRead/17(FIH_Read_EsaEnbl_D_Rq) -> [FIH_Read_EsaEnbl_D_Rq]
  CF054A_FordBlaBoxCanHiSpdRead/18(FIH_Read_EsaOn_B_Rq) -> [FIH_Read_EsaOn_B_Rq]
  CF054A_FordBlaBoxCanHiSpdRead/19(FIH_Read_FIH_Msg_In_1_High) -> [FIH_Read_FIH_Msg_In_1_High]
  CF054A_FordBlaBoxCanHiSpdRead/20(FIH_Read_FIH_Msg_In_1_Low) -> [FIH_Read_FIH_Msg_In_1_Low]
  CF054A_FordBlaBoxCanHiSpdRead/21(FIH_Read_FIH_Msg_In_2_High) -> [FIH_Read_FIH_Msg_In_2_High]
  CF054A_FordBlaBoxCanHiSpdRead/22(FIH_Read_FIH_Msg_In_2_Low) -> [FIH_Read_FIH_Msg_In_2_Low]
  CF054A_FordBlaBoxCanHiSpdRead/23(FIH_Read_FIH_Msg_In_3_High) -> [FIH_Read_FIH_Msg_In_3_High]
  CF054A_FordBlaBoxCanHiSpdRead/24(FIH_Read_FIH_Msg_In_3_Low) -> [FIH_Read_FIH_Msg_In_3_Low]
  CF054A_FordBlaBoxCanHiSpdRead/25(FIH_Read_FIH_Msg_In_4_High) -> [FIH_Read_FIH_Msg_In_4_High]
  CF054A_FordBlaBoxCanHiSpdRead/26(FIH_Read_FIH_Msg_In_4_Low) -> [FIH_Read_FIH_Msg_In_4_Low]
  CF054A_FordBlaBoxCanHiSpdRead/27(FIH_Read_GearLvrPos_D_Actl) -> [FIH_Read_GearLvrPos_D_Actl]
  CF054A_FordBlaBoxCanHiSpdRead/28(FIH_Read_GearPosition) -> [FIH_Read_GearPosition]
  CF054A_FordBlaBoxCanHiSpdRead/29(FIH_Read_GearRvrse_D_Actl) -> [FIH_Read_GearRvrse_D_Actl]
  CF054A_FordBlaBoxCanHiSpdRead/30(FIH_Read_HandsOffCnfm_B_Rq) -> [FIH_Read_HandsOffCnfm_B_Rq]
  CF054A_FordBlaBoxCanHiSpdRead/31(FIH_Read_HitchToVehAxle) -> [FIH_Read_HitchToVehAxle]
  CF054A_FordBlaBoxCanHiSpdRead/32(FIH_Read_Ignition_Status) -> [FIH_Read_Ignition_Status]
  CF054A_FordBlaBoxCanHiSpdRead/33(FIH_Read_LaCurvature_No_Calc) -> [FIH_Read_LaCurvature_No_Calc]
  CF054A_FordBlaBoxCanHiSpdRead/34(FIH_Read_LaRampType_B_Req) -> [FIH_Read_LaRampType_B_Req]
  CF054A_FordBlaBoxCanHiSpdRead/35(FIH_Read_LaRefAng_No_Req) -> [FIH_Read_LaRefAng_No_Req]
  CF054A_FordBlaBoxCanHiSpdRead/36(FIH_Read_LatCtlCurv_NoRate_Actl) -> [FIH_Read_LatCtlCurv_NoRate_Actl]
  CF054A_FordBlaBoxCanHiSpdRead/37(FIH_Read_LatCtlCurv_No_Actl) -> [FIH_Read_LatCtlCurv_No_Actl]
  CF054A_FordBlaBoxCanHiSpdRead/38(FIH_Read_LatCtlPathOffst_L_Actl) -> [FIH_Read_LatCtlPathOffst_L_Actl]
  CF054A_FordBlaBoxCanHiSpdRead/39(FIH_Read_LatCtlPath_An_Actl) -> [FIH_Read_LatCtlPath_An_Actl]
  CF054A_FordBlaBoxCanHiSpdRead/40(FIH_Read_LatCtlPrecision_D_Rq) -> [FIH_Read_LatCtlPrecision_D_Rq]
  CF054A_FordBlaBoxCanHiSpdRead/41(FIH_Read_LatCtlRampType_D_Rq) -> [FIH_Read_LatCtlRampType_D_Rq]
  CF054A_FordBlaBoxCanHiSpdRead/42(FIH_Read_LatCtlRangeMax) -> [FIH_Read_LatCtlRangeMax]
  CF054A_FordBlaBoxCanHiSpdRead/43(FIH_Read_LatCtl_D_Rq) -> [FIH_Read_LatCtl_D_Rq]
  CF054A_FordBlaBoxCanHiSpdRead/44(FIH_Read_LdwActvIntns_D_Req) -> [FIH_Read_LdwActvIntns_D_Req]
  CF054A_FordBlaBoxCanHiSpdRead/45(FIH_Read_LdwActvStats_D_Req) -> [FIH_Read_LdwActvStats_D_Req]
  CF054A_FordBlaBoxCanHiSpdRead/46(FIH_Read_LkaActvStats_D_Req) -> [FIH_Read_LkaActvStats_D_Req]
  CF054A_FordBlaBoxCanHiSpdRead/47(FIH_Read_LsmcBrkDecel_D_Stat) -> [FIH_Read_LsmcBrkDecel_D_Stat]
  CF054A_FordBlaBoxCanHiSpdRead/48(FIH_Read_PrplWhlTot2_Tq_Actl) -> [FIH_Read_PrplWhlTot2_Tq_Actl]
  CF054A_FordBlaBoxCanHiSpdRead/49(FIH_Read_SAPPStatusCoding) -> [FIH_Read_SAPPStatusCoding]
  CF054A_FordBlaBoxCanHiSpdRead/50(FIH_Read_StabCtlBrkActv_B_Actl) -> [FIH_Read_StabCtlBrkActv_B_Actl]
  CF054A_FordBlaBoxCanHiSpdRead/51(FIH_Read_StePinOffst_An_Est) -> [FIH_Read_StePinOffst_An_Est]
  CF054A_FordBlaBoxCanHiSpdRead/52(FIH_Read_StePinOffst_D_Stat) -> [FIH_Read_StePinOffst_D_Stat]
  CF054A_FordBlaBoxCanHiSpdRead/53(FIH_Read_TrlrAidCancl_B_Rq) -> [FIH_Read_TrlrAidCancl_B_Rq]
  CF054A_FordBlaBoxCanHiSpdRead/54(FIH_Read_TrlrAidCtl_U_RqDrv) -> [FIH_Read_TrlrAidCtl_U_RqDrv]
  CF054A_FordBlaBoxCanHiSpdRead/55(FIH_Read_TrlrAidEnbl_D2_Rq) -> [FIH_Read_TrlrAidEnbl_D2_Rq]
  CF054A_FordBlaBoxCanHiSpdRead/56(FIH_Read_TrlrAidSetup_Rq) -> [FIH_Read_TrlrAidSetup_Rq]
  CF054A_FordBlaBoxCanHiSpdRead/57(FIH_Read_TrlrAidSwtch_D_RqDrv) -> [FIH_Read_TrlrAidSwtch_D_RqDrv]
  CF054A_FordBlaBoxCanHiSpdRead/58(FIH_Read_TrlrAidTrgtId) -> [FIH_Read_TrlrAidTrgtId]
  CF054A_FordBlaBoxCanHiSpdRead/59(FIH_Read_TrlrAid_Angle) -> [FIH_Read_TrlrAid_Angle]
  CF054A_FordBlaBoxCanHiSpdRead/60(FIH_Read_TrlrAid_AngleRate) -> [FIH_Read_TrlrAid_AngleRate]
  CF054A_FordBlaBoxCanHiSpdRead/61(FIH_Read_TrlrAid_D2_Stat) -> [FIH_Read_TrlrAid_D2_Stat]
  CF054A_FordBlaBoxCanHiSpdRead/62(FIH_Read_TrlrAid_Mode_Rq) -> [FIH_Read_TrlrAid_Mode_Rq]
  CF054A_FordBlaBoxCanHiSpdRead/63(FIH_Read_TrlrAnOffstDir_Mem) -> [FIH_Read_TrlrAnOffstDir_Mem]
  CF054A_FordBlaBoxCanHiSpdRead/64(FIH_Read_TrlrAxleToBmpr_L_Actl) -> [FIH_Read_TrlrAxleToBmpr_L_Actl]
  CF054A_FordBlaBoxCanHiSpdRead/65(FIH_Read_TrlrBrkActCnnct_B_Actl) -> [FIH_Read_TrlrBrkActCnnct_B_Actl]
  CF054A_FordBlaBoxCanHiSpdRead/66(FIH_Read_TrlrHitYaw_AnRate) -> [FIH_Read_TrlrHitYaw_AnRate]
  CF054A_FordBlaBoxCanHiSpdRead/67(FIH_Read_TrlrHitchYaw_An) -> [FIH_Read_TrlrHitchYaw_An]
  CF054A_FordBlaBoxCanHiSpdRead/68(FIH_Read_TrlrHitchYaw_Stat) -> [FIH_Read_TrlrHitchYaw_Stat]
  CF054A_FordBlaBoxCanHiSpdRead/69(FIH_Read_TrlrIdType_Stat) -> [FIH_Read_TrlrIdType_Stat]
  CF054A_FordBlaBoxCanHiSpdRead/70(FIH_Read_TrlrId_No_Actl) -> [FIH_Read_TrlrId_No_Actl]
  CF054A_FordBlaBoxCanHiSpdRead/71(FIH_Read_TrlrLampCnnct_B_Actl) -> [FIH_Read_TrlrLampCnnct_B_Actl]
  CF054A_FordBlaBoxCanHiSpdRead/72(FIH_Read_TrlrRvrseCancl_Rq) -> [FIH_Read_TrlrRvrseCancl_Rq]
  CF054A_FordBlaBoxCanHiSpdRead/73(FIH_Read_TrlrRvrseEnbl) -> [FIH_Read_TrlrRvrseEnbl]
  CF054A_FordBlaBoxCanHiSpdRead/74(FIH_Read_TrlrRvrseMsgTxt) -> [FIH_Read_TrlrRvrseMsgTxt]
  CF054A_FordBlaBoxCanHiSpdRead/75(FIH_Read_TrlrRvrseOn_Stat) -> [FIH_Read_TrlrRvrseOn_Stat]
  CF054A_FordBlaBoxCanHiSpdRead/76(FIH_Read_TrlrSnsId) -> [FIH_Read_TrlrSnsId]
  CF054A_FordBlaBoxCanHiSpdRead/77(FIH_Read_TrlrTrgtAcquire) -> [FIH_Read_TrlrTrgtAcquire]
  CF054A_FordBlaBoxCanHiSpdRead/78(FIH_Read_TrlrYaw_W) -> [FIH_Read_TrlrYaw_W]
  CF054A_FordBlaBoxCanHiSpdRead/79(FIH_Read_TrlrYaw_W_Qf) -> [FIH_Read_TrlrYaw_W_Qf]
  CF054A_FordBlaBoxCanHiSpdRead/80(FIH_Read_TrnRng) -> [FIH_Read_TrnRng]
  CF054A_FordBlaBoxCanHiSpdRead/81(FIH_Read_TurnLghtSwtch_D_Stat) -> [FIH_Read_TurnLghtSwtch_D_Stat]
  CF054A_FordBlaBoxCanHiSpdRead/82(FIH_Read_VehLatComp_A_Actl) -> [FIH_Read_VehLatComp_A_Actl]
  CF054A_FordBlaBoxCanHiSpdRead/83(FIH_Read_VehLongComp_A_Actl) -> [FIH_Read_VehLongComp_A_Actl]
  CF054A_FordBlaBoxCanHiSpdRead/84(FIH_Read_VehOverGnd_V_Est) -> [FIH_Read_VehOverGnd_V_Est]
  CF054A_FordBlaBoxCanHiSpdRead/85(FIH_Read_VehVTrlrAid_B_Avail) -> [FIH_Read_VehVTrlrAid_B_Avail]
  CF054A_FordBlaBoxCanHiSpdRead/86(FIH_Read_VehVertComp) -> [FIH_Read_VehVertComp]
  CF054A_FordBlaBoxCanHiSpdRead/87(FIH_Read_VehYawComp_W_Actl) -> [FIH_Read_VehYawComp_W_Actl]
  CF054A_FordBlaBoxCanHiSpdRead/88(FIH_Read_VehYaw_W_Actl) -> [FIH_Read_VehYaw_W_Actl]
  CF054A_FordBlaBoxCanHiSpdRead/89(FIH_Read_Veh_V_ActlBrk) -> [FIH_Read_Veh_V_ActlBrk]
  CF054A_FordBlaBoxCanHiSpdRead/90(FIH_Read_WhlDirFl_D_Actl) -> [FIH_Read_WhlDirFl_D_Actl]
  CF054A_FordBlaBoxCanHiSpdRead/91(FIH_Read_WhlDirFr_D_Actl) -> [FIH_Read_WhlDirFr_D_Actl]
  CF054A_FordBlaBoxCanHiSpdRead/92(FIH_Read_WhlDirRl_D_Actl) -> [FIH_Read_WhlDirRl_D_Actl]
  CF054A_FordBlaBoxCanHiSpdRead/93(FIH_Read_WhlDirRr_D_Actl) -> [FIH_Read_WhlDirRr_D_Actl]
  CF054A_FordBlaBoxCanHiSpdRead/94(FIH_Read_WhlFl_W_Meas) -> [FIH_Read_WhlFl_W_Meas]
  CF054A_FordBlaBoxCanHiSpdRead/95(FIH_Read_WhlFr_W_Meas) -> [FIH_Read_WhlFr_W_Meas]
  CF054A_FordBlaBoxCanHiSpdRead/96(FIH_Read_WhlRl_W_Meas) -> [FIH_Read_WhlRl_W_Meas]
  CF054A_FordBlaBoxCanHiSpdRead/97(FIH_Read_WhlRr_W_Meas) -> [FIH_Read_WhlRr_W_Meas]
  CF054A_FordBlaBoxCanHiSpdRead/98(FIH_Read_Whl_Fl_Roll_Cnt) -> [FIH_Read_Whl_Fl_Roll_Cnt]
  CF054A_FordBlaBoxCanHiSpdRead/99(FIH_Read_Whl_Fr_Roll_Cnt) -> [FIH_Read_Whl_Fr_Roll_Cnt]
  CF054A_FordBlaBoxCanHiSpdRead/100(FIH_Read_Whl_Rl_Roll_Cnt) -> [FIH_Read_Whl_Rl_Roll_Cnt]
  CF054A_FordBlaBoxCanHiSpdRead/101(FIH_Read_Whl_Rr_Roll_Cnt) -> [FIH_Read_Whl_Rr_Roll_Cnt]
  CF054A_FordBlaBoxCanHiSpdRead/102(FIH_Read_YawStabilityIndex) -> [FIH_Read_YawStabilityIndex]
  [SemiAutParlParkAgCtrlSts6] -> CF053A_FordBlaBoxEpsRead/27(SemiAutParlParkAgCtrlSts6)
  [FordVehBrkPedlVld] -> CF056A_FordBlaBoxVldRead/65(FordVehBrkPedlVld)
  [VertAccelValid] -> CF056A_FordBlaBoxVldRead/66(VertAccelValid)
  [FilteredVehicleSpeedValid] -> CF056A_FordBlaBoxVldRead/67(FilteredVehicleSpeedValid)
  [EcuId] -> CF062A_FordBlaBoxNvmRead/1(EcuId)
  [FordBlaBoxActvNiblCtrlByte] -> CF062A_FordBlaBoxNvmRead/2(FordBlaBoxActvNiblCtrlByte)
  [FordBlaBoxLaneAssiByte] -> CF062A_FordBlaBoxNvmRead/3(FordBlaBoxLaneAssiByte)
  [FordBlaBoxPullDriftCmpByte] -> CF062A_FordBlaBoxNvmRead/4(FordBlaBoxPullDriftCmpByte)
  [FordBlaBoxTrlrBackupByte] -> CF062A_FordBlaBoxNvmRead/5(FordBlaBoxTrlrBackupByte)
  CF062A_FordBlaBoxNvmRead/1(FIH_ANC_Read_NV_Byte) -> [FIH_ANC_Read_NV_Byte]
  CF062A_FordBlaBoxNvmRead/2(FIH_LA_Read_NV_Byte) -> [FIH_LA_Read_NV_Byte]
  CF062A_FordBlaBoxNvmRead/3(FIH_PDC_Read_NV_Byte) -> [FIH_PDC_Read_NV_Byte]
  CF062A_FordBlaBoxNvmRead/4(FIH_TBA_Read_NV_Byte) -> [FIH_TBA_Read_NV_Byte]
  CF053A_FordBlaBoxEpsRead/30(FIH_Read_TBA_EAC_Status) -> [FIH_Read_TBA_EAC_Status]
  [ExtAgCtrlStsInt] -> CF053A_FordBlaBoxEpsRead/31(ExtAgCtrlStsInt)
  Ground1/1 -> CF053A_FordBlaBoxEpsRead/8(ExtAgCtrlSteerPinionAgVelVld)
